simulink model "opti_debug"  (R2023a)
settings: Solver=FixedStepAuto  StartTime=0.0  StopTime=mdl.rt  RelTol=1e-3
values from neighbouring files (symbols this model uses):
  archived_Eul_XYZ = rst_Eul_XYZ.signals.values    [s4_run.m]    (also in step4_run_v1.m)
  archived_p_raw = rst_p_raw.signals.values    [s4_run.m]    (also in step4_run_v1.m)
  ctr = make_ext_tor_observer(rsim, mdl, ctr)    [s1_setup.m]    (also in setup_controller_with_functions.m = make_controller(); step1_setup.m; step1_setup_v1.m)
  ctr2 = ctr    [s1_setup.m]    (also in step1_setup.m; step1_setup_v1.m)
  lut = gen_lut    [s1_setup.m]    (also in thrust2voltage_lut_20230809.mat = ; thrust2voltage_lut_20230829.mat = )
  mdl = make_model(mdl,rsim)    [s1_setup.m]    (also in setup_controller_with_functions.m = make_model(flight_time); step1_setup.m; step1_setup_v1.m = make_model(flight_time,rsim))
  rbt = make_robot    [s1_setup.m]    (also in setup_controller_with_functions.m = make_robot(); step1_setup.m; step1_setup_v1.m)
  rbt2 = rbt    [s1_setup.m]    (also in step1_setup.m; step1_setup_v1.m)
  rsim = make_robot_simulation()    [setup_controller_with_functions.m]    (also in step1_setup_v1.m = make_simulation(rbt,mdl,rsim))
  sen = make_sensor(mdl,rsim)    [s1_setup.m]
  som = make_somersault(mdl, rsim)    [s1_setup.m]    (also in step1_setup.m)
  Time = logsout.LiveStreamSignals.getElement('voltage').Values.Time    [old_step3_run_controller_v3.m]    (also in post_identify_actuation_response.m = yout(:,1); post_thrust_torque_coefficients.m = yout(:,1))
  traj = make_trajectory(ctr, mdl, rsim)    [s1_setup.m]    (also in step1_setup.m)
undefined symbols (not defined in the file or in its folder): DiscIntNeverNeededParam, Discrete, Standard_Devices, UDP_Protocol
libraries: simulink x27, dspfdesign x12, robotcorelib x7, sldrtlib x7, slrealtimeloglib x1, shared6dof x1, dspsrcs4 x1, uavutilslib x1, ctrlSharedLib x1, dspmathops x1
(part 1 of 4)
settings Model: SimulationMode=external  ExtModeTrigDuration=5000000  Creator=SMRL  LastModifiedBy=SMRL
settings OptimizationCC: DefaultParameterBehavior=Inlined  SimCompilerOptimization=on  AccelVerboseBuild=on
settings HardwareCC: ProdBitPerLong=64  ProdHWDeviceType=Intel->x86-64 (Linux 64)
settings ModelReferenceCC: EnableParallelModelReferenceBuilds=on
settings SFSimCC: SimHardwareAcceleration=native
settings RTWCC: Description=Simulink Desktop Real-Time  SystemTargetFile=sldrt.tlc  TemplateMakefile=sldrt.tmf  RTWCompilerOptimization=on
settings CodeAppCC: MaxIdLength=95
settings SimulinkDesktopRealTimeCC: TargetLibSuffix=_sldrt.a  TargetPreCompLibLocation=C:\Program Files\MATLAB\R2023a\toolbox\sldrt\lib\win64

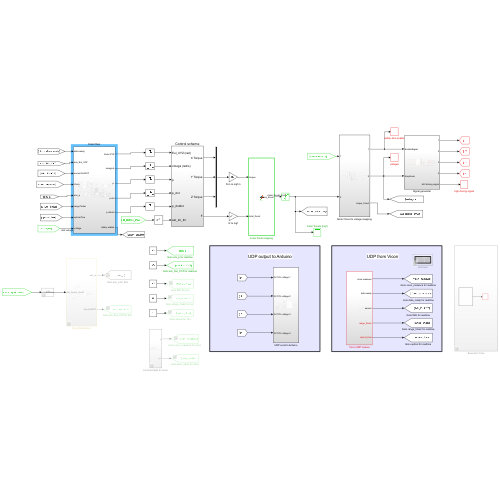
[thumbnail: Simulink's stored preview of the top-level diagram]
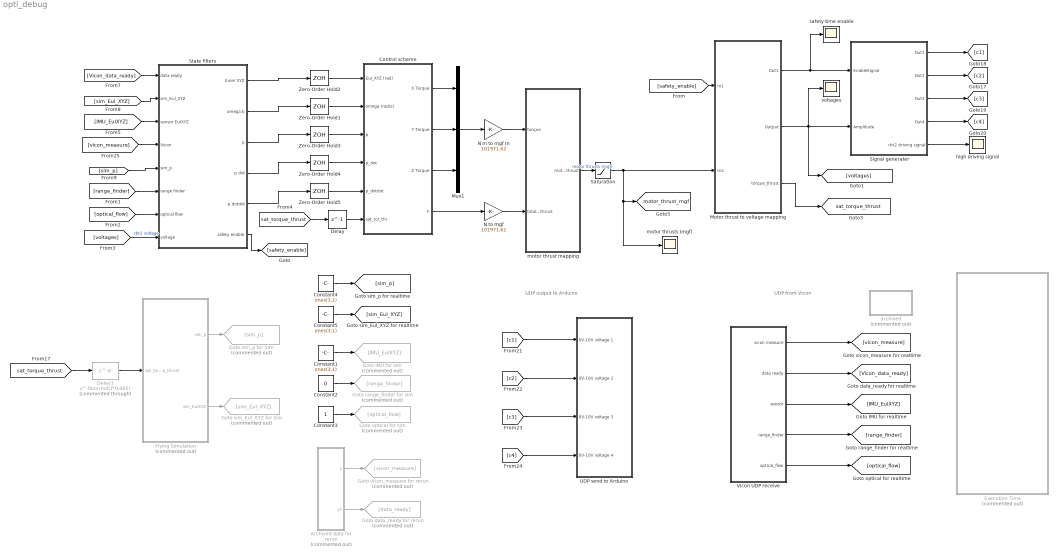
== system opti_debug ==
  note: UDP output to Arduino
  note: UDP from Vicon
  Archived data for rerun : Subsystem  Commented=on
  Constant1 : Constant  Value=ones(3,1)  SampleTime=1/400
  Constant2 : Constant  Value=0  SampleTime=1/400
  Constant3 : Constant  SampleTime=1/400
  Constant4 : Constant  Value=ones(3,1)
  Constant5 : Constant  Value=ones(3,1)
  Control scheme : Subsystem
  Delay : Delay  DelayLength=1  InitialCondition=zeros(4,1)
  Delay1 : Delay  Commented=through  DelayLength=floor(mdl.f*0.005)  InitialCondition=zeros(4,floor(mdl.f*0.005))  SampleTime=mdl.T
  Execution Time : Subsystem  Commented=on
  Flying Simulation : Subsystem  Commented=on
  Goto IMU for sim : Goto  Commented=on  GotoTag=IMU_EulXYZ
  Goto data_ready for rerun : Goto  Commented=on  GotoTag=data_ready
  Goto optical for sim : Goto  Commented=on  GotoTag=optical_flow
  Goto range_finder for sim : Goto  Commented=on  GotoTag=range_finder
  Goto sim_Eul_XYZ for Sim : Goto  Commented=on  GotoTag=sim_Eul_XYZ
  Goto sim_p for Sim : Goto  Commented=on  GotoTag=sim_p
  Goto vicon_measure for rerun : Goto  Commented=on  GotoTag=vicon_measure
  Motor thrust to voltage mapping : Subsystem
  Mux1 : Mux  Inputs=3
  N m to mgf m : Gain  Gain=101971.62
  N to mgf : Gain  Gain=101971.62
  Saturation : Saturate  UpperLimit=1000  LowerLimit=0
  Signal generater : Subsystem
  State filters : Subsystem
  UDP send to Arduino : Subsystem
  Vicon UDP receive : Subsystem
  Zero-Order Hold{1..5} (5 alike) : ZeroOrderHold  SampleTime=mdl.T
  archived : Subsystem  Commented=on
  high driving signal : Scope
  motor thrust mapping : MATLAB Function  TreatAsAtomicUnit=on  SystemSampleTime=mdl.T
  motor thrusts (mgf) : Scope
  safety-time enable : Scope
  voltages : Scope
  tag scope: motor_thrust_mgf=global, sat_torque_thrust=global
  wires:
  motor thrust mapping/1(motors_thrust) -> Saturation/1  "motor thrusts (mgf)"
  Vicon UDP receive/1(vicon measure) -> [vicon_measure]
  Vicon UDP receive/2(data ready) -> [Vicon_data_ready]
  [c1] -> UDP send to Arduino/1(0V-10V voltage 1)
  [c3] -> UDP send to Arduino/3(0V-10V voltage 3)
  [c4] -> UDP send to Arduino/4(0V-10V voltage 4)
  State filters/6(safety enable) -> [safety_enable]
  Control scheme/1(X Torque) -> Mux1/1
  Control scheme/2(Y Torque) -> Mux1/2
  Control scheme/3(Z Torque) -> Mux1/3
  [sat_torque_thrust] -> Delay1/1
  Flying Simulation/2(sim_EulXYZ) -> Goto sim_Eul_XYZ for Sim/1
  Flying Simulation/1(sim_p) -> Goto sim_p for Sim/1
  State filters/1(Euler XYZ) -> Zero-Order Hold2/1
  State filters/2(omega b) -> Zero-Order Hold1/1
  State filters/3("p ") -> Zero-Order Hold3/1
  State filters/4(p dot) -> Zero-Order Hold4/1
  Zero-Order Hold2/1 -> Control scheme/1(Eul_XYZ (rad))
  Zero-Order Hold1/1 -> Control scheme/2(omega (rad/s))
  Zero-Order Hold3/1 -> Control scheme/3(p)
  Zero-Order Hold4/1 -> Control scheme/4(p_dot)
  Zero-Order Hold5/1 -> Control scheme/5(p_dotdot)
  State filters/5(p dotdot) -> Zero-Order Hold5/1
  N m to mgf m/1 -> motor thrust mapping/1(torque)
  N to mgf/1 -> motor thrust mapping/2(total_thrust)
  Constant4/1 -> [sim_p]
  Constant5/1 -> [sim_Eul_XYZ]
  Archived data for rerun/1(y) -> Goto vicon_measure for rerun/1
  Archived data for rerun/2(y1) -> Goto data_ready for rerun/1
  Control scheme/4(" F") -> N to mgf/1
  Mux1/1 -> N m to mgf m/1
  [sat_torque_thrust] -> Delay/1
  Delay/1 -> Control scheme/6(sat_tor_thr)
  Delay1/1 -> Flying Simulation/1(sat_torque_thrust)
  Signal generater/1(Out1) -> [c1]
  Signal generater/2(Out2) -> [c2]
  Signal generater/3(Out3) -> [c3]
  Signal generater/4(Out4) -> [c4]
  Signal generater/5(rbt2 driving signal) -> high driving signal/1
  Motor thrust to voltage mapping/1(Out1) -> Signal generater/1(EnableSignal), safety-time enable/1
  [safety_enable] -> Motor thrust to voltage mapping/1(In1)
  Motor thrust to voltage mapping/2(Output) -> voltages/1, [voltages], Signal generater/2(Amplitude)
  Motor thrust to voltage mapping/3(torque_thrust) -> [sat_torque_thrust]
  Vicon UDP receive/3(sensor) -> [IMU_EulXYZ]
  [c2] -> UDP send to Arduino/2(0V-10V voltage 2)
  Vicon UDP receive/4(range_finder) -> [range_finder]
  [voltages] -> State filters/8(voltage)  "rbt2 voltage"
  [Vicon_data_ready] -> State filters/1(data ready)
  [sim_Eul_XYZ] -> State filters/2(sim_Eul_XYZ)
  [IMU_EulXYZ] -> State filters/3(sensor EulXYZ)
  [vicon_measure] -> State filters/4(Vicon)
  [sim_p] -> State filters/5(sim_p)
  [range_finder] -> State filters/6(range finder)
  Vicon UDP receive/5(optical_flow) -> [optical_flow]
  [optical_flow] -> State filters/7(optical flow)
  Constant2/1 -> Goto range_finder for sim/1
  Constant1/1 -> Goto IMU for sim/1
  Constant3/1 -> Goto optical for sim/1
  Saturation/1 -> Motor thrust to voltage mapping/2(In2), motor thrusts (mgf)/1, [motor_thrust_mgf]

== system opti_debug/Archived data for rerun ==
  MATLAB Function1 : MATLAB Function  TreatAsAtomicUnit=on
  MATLAB Function2 : MATLAB Function  TreatAsAtomicUnit=on
  Scope1 : Scope
  Scope2 : Scope
  Scope3 : Scope
  time1 : Subsystem
  y : Outport
  y1 : Outport  Port=2
  wires:
  MATLAB Function2/1(y) -> y/1, Scope1/1
  time1/1(index) -> Scope2/1, MATLAB Function2/1(t), MATLAB Function1/1(t)
  MATLAB Function1/1(y) -> y1/1, Scope3/1

== system opti_debug/Control scheme ==
  Eul_XYZ (rad) : Inport
  omega (rad/s) : Inport  Port=2
  p : Inport  Port=3
  p_dot : Inport  Port=4
  p_dotdot : Inport  Port=5
  sat_tor_thr : Inport  Port=6
  Coordinate Transformation Conversion : robotcorelib/Coordinate Transformation Conversion  InputRepresentation=Euler Angles  InputEulerSequence=XYZ  ShowTrVecInputPort=on  OutputRepresentation=Rotation Matrix  OutputEulerSequence=ZYX  ShowTrVecOutputPort=on  SimulateUsing=Interpreted execution
  Delay : Delay  DelayLength=1  InitialCondition=1
  Delay1 : Delay  DelayLength=1  InitialCondition=zeros(3,1)
  Subsystem : Subsystem
  adaptive setpoint rd : MATLAB Function  TreatAsAtomicUnit=on  SystemSampleTime=mdl.T
  all states : Scope  NumInputPorts=4
  attitude and thrust controller : Subsystem
  observer : Subsystem  Commented=on
  p vs p_des : Scope  NumInputPorts=2
  saturation : MATLAB Function  TreatAsAtomicUnit=on
  time : Subsystem
  unsat thrust : Scope
  unsat torque : Scope  NumInputPorts=3
  X Torque : Outport
  Y Torque : Outport  Port=2
  Z Torque : Outport  Port=3
  " F" : Outport  Port=4
  wires:
  Eul_XYZ (rad)/1 -> Coordinate Transformation Conversion/1
  omega (rad/s)/1 -> all states/4, attitude and thrust controller/5(Omega)
  saturation/1(X_roll) -> X Torque/1
  saturation/2(Y_pitch) -> Y Torque/1
  saturation/3(Z_yaw) -> Z Torque/1
  saturation/4(Force) -> " F"/1
  attitude and thrust controller/4(F) -> saturation/4(F), unsat thrust/1
  adaptive setpoint rd/1(rd) -> p vs p_des/2, attitude and thrust controller/6(rd)  "rd"
  adaptive setpoint rd/3(rd_dd) -> attitude and thrust controller/8(rd_dd)
  adaptive setpoint rd/4(rd_ddd) -> attitude and thrust controller/9(rd_ddd)
  adaptive setpoint rd/5(rd_dddd) -> attitude and thrust controller/10(rd_dddd)
  time/1(real times) -> adaptive setpoint rd/2(time)
  attitude and thrust controller/3(torque_z) -> saturation/3(z_yaw), unsat torque/3
  attitude and thrust controller/2(torque_y) -> saturation/2(y_pitch), unsat torque/2
  attitude and thrust controller/1(torque_x) -> unsat torque/1, saturation/1(x_roll)
  adaptive setpoint rd/7(id_out) -> Delay/1
  Delay/1 -> adaptive setpoint rd/4(id_in)
  Coordinate Transformation Conversion/1 -> all states/3, attitude and thrust controller/4(R)  "rotm"
  p_dot/1 -> all states/2, attitude and thrust controller/2(r_dot)
  p_dotdot/1 -> attitude and thrust controller/3(r_dotdot)
  p/1 -> adaptive setpoint rd/1(r), p vs p_des/1, attitude and thrust controller/1(r), all states/1
  adaptive setpoint rd/6(init_r_out) -> Delay1/1
  Delay1/1 -> adaptive setpoint rd/3(init_r_in)
  sat_tor_thr/1 -> attitude and thrust controller/11(sat_tor_thr)
  adaptive setpoint rd/2(rd_d) -> Subsystem/1(In1)
  Subsystem/1(Out1) -> attitude and thrust controller/7(rd_d)

== system opti_debug/Execution Time ==
  Execution Time : sldrtlib/Target Profiling/Execution Time  ShowTaskTimes=off
  high execution time : Scope
  wires:
  Execution Time/1 -> high execution time/1

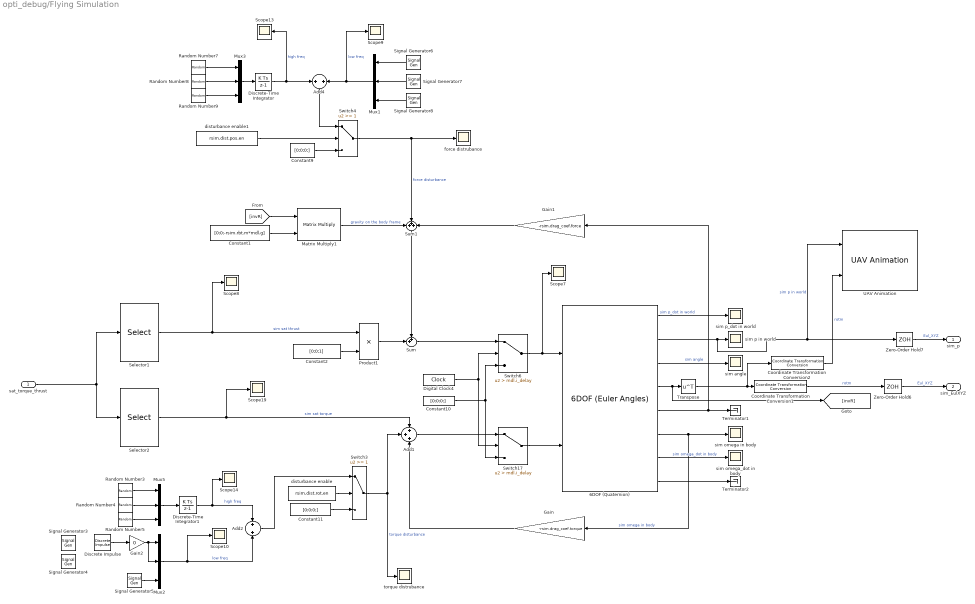
== system opti_debug/Flying Simulation ==
  sat_torque_thrust : Inport
  6DOF (Quaternion) : shared6dof/6DOF (Euler Angles)  units=Metric (MKS)  mtype=Fixed  rep=Quaternion  xme_0=rsim.p0  Vm_0=rsim.v0_b  eul_0=[rsim.Eul_XYZ.x rsim.Eul_XYZ.y rsim.Eul_XYZ.z]  pm_0=rsim.w0  mass_0=rsim.rbt.m  mass_e=0.5  mass_f=2.0  inertia=diag([rsim.rbt.ixx, rsim.rbt.iyy, rsim.rbt.izz])  inertia_e=eye(3)  inertia_f=2*eye(3)  k_quat=1.0  vre_flag=on  abi_flag=off  aMode=0  xme_statename=''  Vm_statename=''  eul_statename=''  quat_statename=''  pm_statename=''  mass_statename=''
      settings: LibrarySourceBlock=aerolib6dof2/6DOF (Quaternion)
  Add1 : Sum  Inputs=+++
  Add2 : Sum
  Add4 : Sum
  Constant1 : Constant  Value=[0;0;-rsim.rbt.m*mdl.g]
  Constant10 : Constant  Value=[0;0;0;]
  Constant11 : Constant  Value=[0;0;0;]
  Constant2 : Constant  Value=[0;0;1]
  Constant9 : Constant  Value=[0;0;0;]
  Coordinate Transformation Conversion1 : robotcorelib/Coordinate Transformation Conversion  InputRepresentation=Rotation Matrix  InputEulerSequence=XYZ  ShowTrVecInputPort=on  OutputRepresentation=Euler Angles  OutputEulerSequence=XYZ  ShowTrVecOutputPort=on  SimulateUsing=Interpreted execution
  Coordinate Transformation Conversion2 : robotcorelib/Coordinate Transformation Conversion  InputRepresentation=Rotation Matrix  InputEulerSequence=XYZ  ShowTrVecInputPort=on  OutputRepresentation=Quaternion  OutputEulerSequence=XYZ  ShowTrVecOutputPort=on  SimulateUsing=Interpreted execution
  Digital Clock4 : DigitalClock  SampleTime=1/2000
  Discrete Impulse : dspsrcs4/Discrete  Impulse  Delay=mdl.f*3.1  SampleTime=mdl.T  FrameSample=1  OutputFrames=off  dataType=double  isSigned=on  wordLen=16  udDataType=sfix(16)  fracBitsMode=Best precision  numFracBits=15  OutDataTypeStr=double  LastOutDataTypeStr=double
  Discrete-Time Integrator : DiscreteIntegrator  InitialCondition=[rsim.dist.x.mean; rsim.dist.y.mean; rsim.dist.z.mean]  SampleTime=mdl.T  ICPrevOutput=DiscIntNeverNeededParam  ICPrevScaledInput=DiscIntNeverNeededParam
  Discrete-Time Integrator1 : DiscreteIntegrator  InitialCondition=[rsim.dist.wx.mean; rsim.dist.wy.mean; rsim.dist.wz.mean]  SampleTime=mdl.T  ICPrevOutput=DiscIntNeverNeededParam  ICPrevScaledInput=DiscIntNeverNeededParam
  Gain : Gain  Gain=-rsim.drag_coef.torque
  Gain1 : Gain  Gain=-rsim.drag_coef.force
  Gain2 : Gain  Gain=0
  Matrix Multiply1 : Product  Multiplication=Matrix(*)
  Mux{1..3,5} (4 alike) : Mux  Inputs=3
  Product1 : Product
  Random Number3 : RandomNumber  Variance=rsim.dist.wx.var  Seed=rsim.dist.wx.seed  SampleTime=1/2000
  Random Number4 : RandomNumber  Variance=rsim.dist.wy.var  Seed=rsim.dist.wy.seed  SampleTime=1/2000
  Random Number5 : RandomNumber  Variance=rsim.dist.wz.var  Seed=rsim.dist.wz.seed  SampleTime=1/2000
  Random Number7 : RandomNumber  Variance=rsim.dist.x.var  Seed=rsim.dist.x.seed  SampleTime=mdl.T
  Random Number8 : RandomNumber  Variance=rsim.dist.y.var  Seed=rsim.dist.y.seed  SampleTime=mdl.T
  Random Number9 : RandomNumber  Variance=rsim.dist.z.var  Seed=rsim.dist.z.seed  SampleTime=mdl.T
  Scope{7..10,13..14,19} (7 alike) : Scope
  Selector1 : Selector  InputPortWidth=4  IndexOptions=Index vector (dialog)  Indices=[4]  OutputSizes=1
  Selector2 : Selector  InputPortWidth=4  IndexOptions=Index vector (dialog)  Indices=[1:3]  OutputSizes=1
  Signal Generator3 : SignalGenerator  WaveForm=square  Amplitude=2e-5  Frequency=0.1618
  Signal Generator4 : SignalGenerator  WaveForm=square  Amplitude=0e-5  Frequency=0.162
  Signal Generator5 : SignalGenerator  Amplitude=-30e-8  Frequency=0.4
  Signal Generator6 : SignalGenerator  WaveForm=square  Amplitude=0  Frequency=0.1
  Signal Generator7 : SignalGenerator  WaveForm=square  Amplitude=0  Frequency=0.5
  Signal Generator8 : SignalGenerator  WaveForm=square  Amplitude=0  Frequency=0.5
  Sum : Sum  Inputs=++|
  Sum1 : Sum  Inputs=+++
  Switch17 : Switch  Criteria=u2 > Threshold  Threshold=mdl.i_delay  SaturateOnIntegerOverflow=off  InputSameDT=off
  Switch3 : Switch  Threshold=1  SaturateOnIntegerOverflow=off  InputSameDT=off
  Switch4 : Switch  Threshold=1  SaturateOnIntegerOverflow=off  InputSameDT=off
  Switch6 : Switch  Criteria=u2 > Threshold  Threshold=mdl.i_delay  SaturateOnIntegerOverflow=off  InputSameDT=off
  Terminator1 : Terminator
  Terminator2 : Terminator
  Transpose : Math  Operator=transpose  SignedPower=on
  UAV Animation : uavutilslib/UAV Animation  UAVType=Multirotor  UAVSize=0.1  InertialZDirection=Up  SampleTime=1/100
  Zero-Order Hold6 : ZeroOrderHold  SampleTime=1/400
  Zero-Order Hold7 : ZeroOrderHold  SampleTime=1/400
  disturbance enable : Constant  Value=rsim.dist.rot.en
  disturbance enable1 : Constant  Value=rsim.dist.pos.en
  force distrubance : Scope
  sim angle : Scope
  sim omega in body : Scope
  sim omega_dot in body : Scope
  sim p in world : Scope
  sim p_dot in world : Scope
  torque distrubance : Scope
  sim_p : Outport
  sim_EulXYZ : Outport  Port=2
  wires:
  Random Number5/1 -> Mux5/3
  disturbance enable/1 -> Switch3/2
  Mux5/1 -> Discrete-Time Integrator1/1
  Digital Clock4/1 -> Switch6/2, Switch17/2
  Constant11/1 -> Switch3/3
  Constant2/1 -> Product1/2
  Constant1/1 -> Matrix Multiply1/2
  Random Number3/1 -> Mux5/1
  Matrix Multiply1/1 -> Sum1/1  "gravity on the body frame"
  disturbance enable1/1 -> Switch4/2
  Random Number4/1 -> Mux5/2
  Switch3/1 -> Add1/2, torque distrubance/1  "torque disturbance"
  Constant9/1 -> Switch4/3
  [invR] -> Matrix Multiply1/1
  Constant10/1 -> Switch6/3, Switch17/3
  Sum1/1 -> Sum/1
  Sum/1 -> Switch6/1
  Switch4/1 -> Sum1/2, force distrubance/1  "force disturbance"
  Product1/1 -> Sum/2
  Add1/1 -> Switch17/1
  Switch6/1 -> Scope7/1, 6DOF (Quaternion)/1
  Switch17/1 -> 6DOF (Quaternion)/2
  6DOF (Quaternion)/1 -> sim p_dot in world/1  "sim p_dot in world"
  6DOF (Quaternion)/2 -> UAV Animation/1, Zero-Order Hold7/1, sim p in world/1  "sim p in world"
  6DOF (Quaternion)/3 -> sim angle/1  "sim angle"
  6DOF (Quaternion)/4 -> [invR], Transpose/1
  6DOF (Quaternion)/5 -> Gain1/1, Terminator1/1
  6DOF (Quaternion)/6 -> Gain/1, sim omega in body/1  "sim omega in body"
  6DOF (Quaternion)/7 -> sim omega_dot in body/1  "sim omega_dot in body"
  6DOF (Quaternion)/8 -> Terminator2/1
  Transpose/1 -> Coordinate Transformation Conversion2/1, Coordinate Transformation Conversion1/1
  Zero-Order Hold6/1 -> sim_EulXYZ/1  "Eul_XYZ"
  Coordinate Transformation Conversion1/1 -> Zero-Order Hold6/1  "rotm"
  Zero-Order Hold7/1 -> sim_p/1  "Eul_XYZ"
  Mux2/1 -> Scope10/1, Add2/2  "low freq"
  Signal Generator5/1 -> Mux2/3
  sat_torque_thrust/1 -> Selector1/1, Selector2/1
  Selector1/1 -> Scope8/1, Product1/1  "sim sat thrust"
  Selector2/1 -> Scope19/1, Add1/1  "sim sat torque"
  Random Number7/1 -> Mux3/1
  Mux3/1 -> Discrete-Time Integrator/1
  Random Number8/1 -> Mux3/2
  Random Number9/1 -> Mux3/3
  Discrete-Time Integrator/1 -> Add4/1, Scope13/1  "high freq"
  Mux1/1 -> Scope9/1, Add4/2  "low freq"
  Signal Generator8/1 -> Mux1/3
  Signal Generator7/1 -> Mux1/2
  Signal Generator6/1 -> Mux1/1
  Add4/1 -> Switch4/1
  Discrete-Time Integrator1/1 -> Add2/1, Scope14/1  "high freq"
  Add2/1 -> Switch3/1
  Coordinate Transformation Conversion2/1 -> UAV Animation/2  "rotm"
  Gain/1 -> Add1/3
  Gain1/1 -> Sum1/3
  Discrete Impulse/1 -> Gain2/1
  Gain2/1 -> Mux2/2, Mux2/1

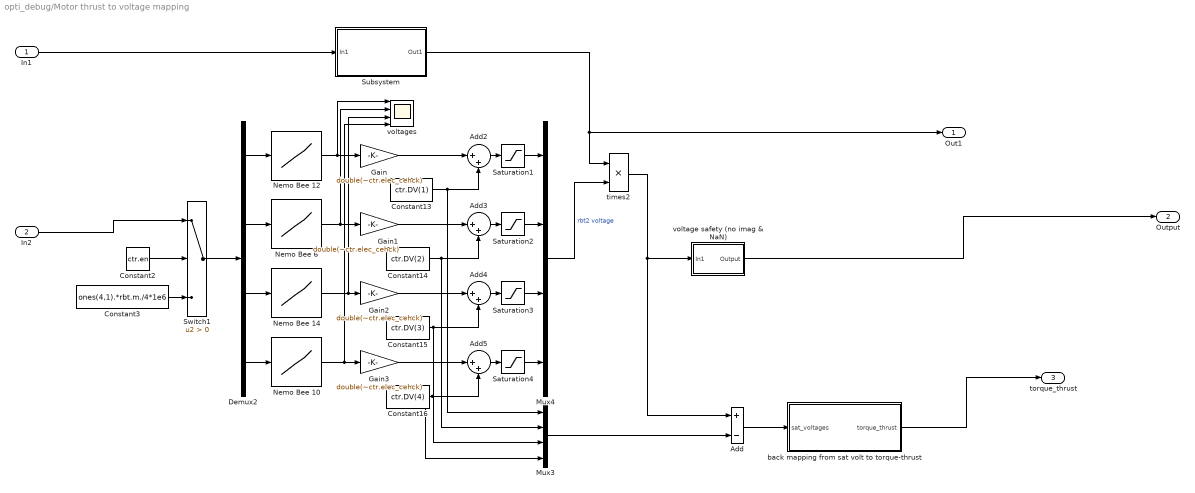
== system opti_debug/Motor thrust to voltage mapping ==
  In1 : Inport
  In2 : Inport  Port=2
  Add : Sum  Inputs=+-
  Add{2..5} (4 alike) : Sum  Inputs=|++
  Constant13 : Constant  Value=ctr.DV(1)
  Constant14 : Constant  Value=ctr.DV(2)
  Constant15 : Constant  Value=ctr.DV(3)
  Constant16 : Constant  Value=ctr.DV(4)
  Constant2 : Constant  Value=ctr.en
  Constant3 : Constant  Value=ones(4,1).*rbt.m./4*1e6
  Demux2 : Demux
  Gain{,1..3} (4 alike) : Gain  Gain=double(~ctr.elec_cehck)
  Mux3 : Mux
  Mux4 : Mux
  Nemo Bee 10 : Lookup_n-D  NumberOfTableDimensions=1  BreakpointsForDimension1=lut.T4  Table=lut.v4  InternalRulePriority=Speed  RndMeth=Simplest
  Nemo Bee 12 : Lookup_n-D  NumberOfTableDimensions=1  BreakpointsForDimension1=lut.T1  Table=lut.v1  InternalRulePriority=Speed  RndMeth=Simplest
  Nemo Bee 14 : Lookup_n-D  NumberOfTableDimensions=1  BreakpointsForDimension1=lut.T3  Table=lut.v3  InternalRulePriority=Speed  RndMeth=Simplest
  Nemo Bee 6 : Lookup_n-D  NumberOfTableDimensions=1  BreakpointsForDimension1=lut.T2  Table=lut.v2  InternalRulePriority=Speed  RndMeth=Simplest
  Saturation1 : Saturate  UpperLimit=ctr.safety.volt(1)  LowerLimit=0
  Saturation2 : Saturate  UpperLimit=ctr.safety.volt(2)  LowerLimit=0
  Saturation3 : Saturate  UpperLimit=ctr.safety.volt(3)  LowerLimit=0
  Saturation4 : Saturate  UpperLimit=ctr.safety.volt(4)  LowerLimit=0
  Subsystem : Subsystem
  Switch1 : Switch  Criteria=u2 > Threshold  SaturateOnIntegerOverflow=off  InputSameDT=off
  back mapping from sat volt to torque-thrust : Subsystem
  times2 : Product  RndMeth=Zero
  voltage safety (no imag & NaN) : Subsystem
  voltages : Scope  NumInputPorts=4
  Out1 : Outport
  Output : Outport  Port=2
  torque_thrust : Outport  Port=3
  wires:
  Add4/1 -> Saturation3/1
  Nemo Bee 6/1 -> voltages/2, Gain1/1
  Gain1/1 -> Add3/1
  Add2/1 -> Saturation1/1
  Saturation4/1 -> Mux4/4
  Demux2/1 -> Nemo Bee 12/1
  Constant3/1 -> Switch1/3
  In2/1 -> Switch1/1
  Add5/1 -> Saturation4/1
  Add/1 -> back mapping from sat volt to torque-thrust/1(sat_voltages)
  Gain/1 -> Add2/1
  Constant2/1 -> Switch1/2
  Nemo Bee 12/1 -> voltages/1, Gain/1
  Mux3/1 -> Add/2
  Constant13/1 -> Mux3/1, Add2/2
  Saturation2/1 -> Mux4/2
  Nemo Bee 10/1 -> voltages/4, Gain3/1
  back mapping from sat volt to torque-thrust/1(torque_thrust) -> torque_thrust/1
  Demux2/2 -> Nemo Bee 6/1
  Constant14/1 -> Mux3/2, Add3/2
  Mux4/1 -> times2/2  "rbt2 voltage"
  Demux2/4 -> Nemo Bee 10/1
  Add3/1 -> Saturation2/1
  times2/1 -> Add/1, voltage safety (no imag & NaN)/1(In1)
  In1/1 -> Subsystem/1(In1)
  Switch1/1 -> Demux2/1
  Constant16/1 -> Mux3/4, Add5/2
  Demux2/3 -> Nemo Bee 14/1
  Nemo Bee 14/1 -> voltages/3, Gain2/1
  Subsystem/1(Out1) -> Out1/1, times2/1
  Gain3/1 -> Add5/1
  Gain2/1 -> Add4/1
  Constant15/1 -> Mux3/3, Add4/2
  Saturation3/1 -> Mux4/3
  Saturation1/1 -> Mux4/1
  voltage safety (no imag & NaN)/1(Output) -> Output/1

== system opti_debug/Signal generater ==
  EnableSignal : Inport
  Amplitude : Inport  Port=2
  Demux4 : Demux
  Flapping Freq (Hz) : Constant  Value=ctr.freq_vec  VectorParams1D=off  SampleTime=mdl.T_high
  Mux7 : Mux
  c1 (JP1) : Gain  Gain=0.9739
  c2 (B1) : Gain  Gain=0.9947
  c3 (W1)1 : Gain  Gain=0.9769
  c4 (JP2) : Gain  Gain=0.9910
  safety voltage : Constant  Value=ctr.safety.volt  SampleTime=mdl.T_high
  signal generator1 : Subsystem  SystemSampleTime=mdl.T_high
  signal safety (no imag & NaN) : Subsystem
  Out1 : Outport
  Out2 : Outport  Port=2
  Out3 : Outport  Port=3
  Out4 : Outport  Port=4
  rbt2 driving signal : Outport  Port=5
  wires:
  Mux7/1 -> rbt2 driving signal/1, signal safety (no imag & NaN)/1(In1)  "rbt2 driving signal"
  signal generator1/1(D2A DriveSignal 1) -> Mux7/1
  safety voltage/1 -> signal generator1/2(safety voltage)
  signal safety (no imag & NaN)/1(Output) -> Demux4/1
  Demux4/3 -> c3 (W1)1/1
  Demux4/1 -> c1 (JP1)/1
  Demux4/2 -> c2 (B1)/1
  signal generator1/2(D2A DriveSignal 2) -> Mux7/2
  Demux4/4 -> c4 (JP2)/1
  Flapping Freq (Hz)/1 -> signal generator1/3(frequency_vec (hz))
  signal generator1/3(D2A DriveSignal 3) -> Mux7/3
  signal generator1/4(D2A DriveSignal 4) -> Mux7/4
  EnableSignal/1 -> signal generator1/1(EnableSignal)
  c4 (JP2)/1 -> Out4/1
  c1 (JP1)/1 -> Out1/1
  c2 (B1)/1 -> Out2/1
  c3 (W1)1/1 -> Out3/1
  Amplitude/1 -> signal generator1/4(Amplitude)

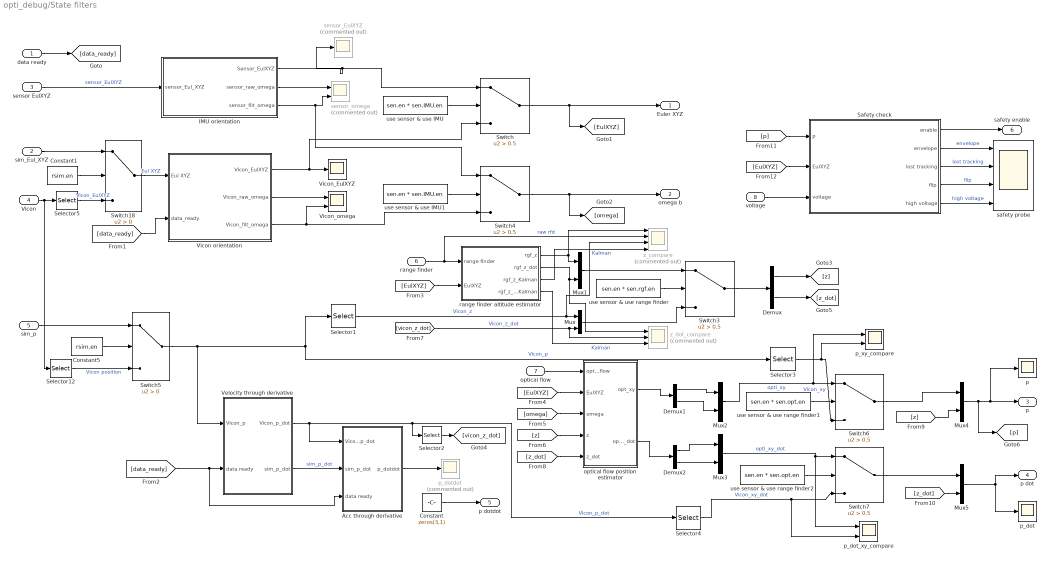
== system opti_debug/State filters ==
  data ready : Inport
  sim_Eul_XYZ : Inport  Port=2
  sensor EulXYZ : Inport  Port=3
  Vicon : Inport  Port=4
  sim_p : Inport  Port=5
  range finder : Inport  Port=6
  optical flow : Inport  Port=7
  voltage : Inport  Port=8
  Acc through derivative : Subsystem
  Constant : Constant  Value=zeros(3,1)
  Constant1 : Constant  Value=rsim.en
  Constant5 : Constant  Value=rsim.en
  Demux : Demux  Outputs=2
  Demux1 : Demux  Outputs=2
  Demux2 : Demux  Outputs=2
  IMU orientation : Subsystem
  Mux{,1..5} (6 alike) : Mux  Inputs=2
  Safety check : Subsystem  SystemSampleTime=mdl.T
  Selector1 : Selector  InputPortWidth=3  IndexOptions=Index vector (dialog)  Indices=[3]  OutputSizes=1
  Selector12 : Selector  InputPortWidth=6  IndexOptions=Index vector (dialog)  Indices=[1:3]  OutputSizes=1
  Selector2 : Selector  InputPortWidth=3  IndexOptions=Index vector (dialog)  Indices=[3]  OutputSizes=1
  Selector3 : Selector  InputPortWidth=3  IndexOptions=Index vector (dialog)  Indices=[1 2]  OutputSizes=1
  Selector4 : Selector  InputPortWidth=3  IndexOptions=Index vector (dialog)  Indices=[1 2]  OutputSizes=1
  Selector5 : Selector  InputPortWidth=6  IndexOptions=Index vector (dialog)  Indices=[4:6]  OutputSizes=1
  Switch{,3..4,6..7} (5 alike) : Switch  Criteria=u2 > Threshold  Threshold=0.5  SaturateOnIntegerOverflow=off  InputSameDT=off
  Switch18 : Switch  Criteria=u2 > Threshold  SaturateOnIntegerOverflow=off  InputSameDT=off
  Switch5 : Switch  Criteria=u2 > Threshold  SaturateOnIntegerOverflow=off  InputSameDT=off
  Velocity through derivative : Subsystem
  Vicon orientation : Subsystem
  Vicon_EulXYZ : Scope
  Vicon_omega : Scope  NumInputPorts=2
  optical flow position estimator : Subsystem
  p : Scope
  p_dot : Scope
  p_dot_xy_compare : Scope  NumInputPorts=2
  p_dotdot : Scope  Commented=on
  p_xy_compare : Scope  NumInputPorts=2
  range finder altitude estimator : Subsystem
  safety probe : Scope  NumInputPorts=4
  sensor_EulXYZ : Scope  Commented=on
  sensor_omega : Scope  Commented=on  NumInputPorts=2
  use sensor & use IMU : Constant  Value=sen.en * sen.IMU.en
  use sensor & use IMU1 : Constant  Value=sen.en * sen.IMU.en
  use sensor & use range finder : Constant  Value=sen.en * sen.rgf.en
  use sensor & use range finder1 : Constant  Value=sen.en * sen.opt.en
  use sensor & use range finder2 : Constant  Value=sen.en * sen.opt.en
  z_compare : Scope  Commented=on  NumInputPorts=4
  z_dot_compare : Scope  Commented=on  NumInputPorts=3
  Euler XYZ : Outport
  omega b : Outport  Port=2
  "p " : Outport  Port=3
  p dot : Outport  Port=4
  p dotdot : Outport  Port=5
  safety enable : Outport  Port=6
  wires:
  Switch5/1 -> Velocity through derivative/1(Vicon_p), Selector1/1, Selector3/1  "Vicon_p"
  Constant1/1 -> Switch18/2
  Vicon/1 -> Selector12/1, Selector5/1
  data ready/1 -> [data_ready]
  sim_p/1 -> Switch5/1
  sim_Eul_XYZ/1 -> Switch18/1
  Safety check/1(enable) -> safety enable/1
  Safety check/2(envelope) -> safety probe/1  "envelope"
  Safety check/3(lost tracking) -> safety probe/2  "lost tracking"
  Safety check/4(flip) -> safety probe/3  "flip"
  Safety check/5(high voltage) -> safety probe/4  "high voltage"
  voltage/1 -> Safety check/3(voltage)
  use sensor & use IMU/1 -> Switch/2
  Switch/1 -> [EulXYZ], Euler XYZ/1
  Switch4/1 -> omega b/1, [omega]
  use sensor & use IMU1/1 -> Switch4/2
  Constant5/1 -> Switch5/2
  range finder/1 -> range finder altitude estimator/1(range finder), z_compare/2  "raw rfd"
  optical flow/1 -> optical flow position estimator/1(optical flow)
  optical flow position estimator/1(opt_xy) -> Demux1/1
  [EulXYZ] -> range finder altitude estimator/2(EulXYZ)
  use sensor & use range finder/1 -> Switch3/2
  [EulXYZ] -> optical flow position estimator/2(EulXYZ)
  [omega] -> optical flow position estimator/3(omega)
  optical flow position estimator/2(opt_xy_dot) -> Demux2/1
  Selector2/1 -> [vicon_z_dot]
  [vicon_z_dot] -> z_dot_compare/2, Mux/2  "Vicon_z_dot"
  Selector1/1 -> z_compare/3, Mux/1  "Vicon_z"
  Mux/1 -> Switch3/3
  range finder altitude estimator/1(rgf_z) -> z_compare/1, Mux1/1
  range finder altitude estimator/2(rgf_z_dot) -> z_dot_compare/1, Mux1/2
  Mux1/1 -> Switch3/1
  Switch3/1 -> Demux/1
  Demux/1 -> [z]
  Demux/2 -> [z_dot]
  [z] -> optical flow position estimator/4(z)
  Demux1/1 -> Mux2/1
  Demux1/2 -> Mux2/2
  Demux2/2 -> Mux3/2
  Demux2/1 -> Mux3/1
  use sensor & use range finder1/1 -> Switch6/2
  Mux2/1 -> p_xy_compare/1, Switch6/1  "opti_xy"
  use sensor & use range finder2/1 -> Switch7/2
  Mux3/1 -> p_dot_xy_compare/1, Switch7/1  "opti_xy_dot"
  Mux5/1 -> p dot/1, p_dot/1
  [p] -> Safety check/1(p)
  [EulXYZ] -> Safety check/2(EulXYZ)
  IMU orientation/1(Sensor_EulXYZ) -> Switch/1, sensor_EulXYZ/1
  IMU orientation/3(sensor_filt_omega) -> sensor_omega/2, Switch4/1
  sensor EulXYZ/1 -> IMU orientation/1(sensor_Eul_XYZ)  "sensor_EulXYZ"
  IMU orientation/2(sensor_raw_omega) -> sensor_omega/1
  Vicon orientation/1(Vicon_EulXYZ) -> Switch/3, Vicon_EulXYZ/1
  Vicon orientation/3(Vicon_filt_omega) -> Switch4/3, Vicon_omega/2
  Switch18/1 -> Vicon orientation/1(Eul XYZ)  "Eul XYZ"
  Vicon orientation/2(Vicon_raw_omega) -> Vicon_omega/1
  Constant/1 -> p dotdot/1
  Velocity through derivative/1(Vicon_p_dot) -> Selector4/1, Selector2/1, Acc through derivative/1(Vicon_p_dot)  "Vicon_p_dot"
  [data_ready] -> Acc through derivative/3(data ready), Velocity through derivative/2(data ready)
  Velocity through derivative/2(sim_p_dot) -> Acc through derivative/2(sim_p_dot)  "sim_p_dot"
  Acc through derivative/1(p_dotdot) -> p_dotdot/1
  [data_ready] -> Vicon orientation/2(data_ready)
  Selector3/1 -> p_xy_compare/2, Switch6/3  "Vicon_xy"
  [z] -> Mux4/2
  Switch6/1 -> Mux4/1
  Mux4/1 -> [p], "p "/1, p/1
  Selector4/1 -> p_dot_xy_compare/2, Switch7/3  "Vicon_xy_dot"
  [z_dot] -> Mux5/2
  Switch7/1 -> Mux5/1
  range finder altitude estimator/3(rgf_z_Kalman) -> z_compare/4  "Kalman"
  range finder altitude estimator/4(rgf_z_dot_Kalman) -> z_dot_compare/3  "Kalman"
  Selector12/1 -> Switch5/3  "Vicon position"
  Selector5/1 -> Switch18/3  "Vicon_EulXYZ"
  [z_dot] -> optical flow position estimator/5(z_dot)

== system opti_debug/UDP send to Arduino ==
  0V-10V voltage 1 : Inport
  0V-10V voltage 2 : Inport  Port=2
  0V-10V voltage 3 : Inport  Port=3
  0V-10V voltage 4 : Inport  Port=4
  Digital Clock : DigitalClock  SampleTime=1/10000
  Packet Output : sldrtlib/Packet Output  SampleTime=1/10000  MaxMissedTicks=100  ShowMissedTicks=off  YieldWhenWaiting=off  DrvName=Standard_Devices/UDP_Protocol  DrvAddress=22099  DrvOptions=[0 25000 49 54 57 46 50 53 52 46 49 48 51 46 52 50 0 0 0 0 0 0 0 0 0 0 0 0 0 0 0 0 0 0 0 0 0 0 0 0 0 0 0 0 0 0 0 0 0 0 0 0 0 0 0 0 0 0 0 0 0 0 0 0 0 0 0 0 0 0 0 0 0 0 0 0 0 0 0 0 0 0 0 0 0 0 0 0 0 0 0 0 0 0 0 0 0 0 0 0 0 0 0 0 0 0 0 0 0 0 0 0 0 0 0 0 0 0 0 0 0 0 0 0 0 0 0 0 0 0 0 0 0 0 0 0 0 0 0 0 0 0 0 0 0 0 0 0 0 0 0 0 0 0 0 0 0 0 0 0 0 0 0 0 0 0 0 0 0 0 0 0 0 0 0 0 0 0 0 0 0 0 0 0 0 0 0 0 0 0 0 0 0 0 0 0 0 0 0 0 0 0 0 0 0 0 0 0 0 0 0 0 0 0 0 0 0 0 0 0 0 0 0 0 0 0 0 0 0 0 0 0 0 0 0 0 0 0 0 0 0 0 0 0 0 0 0 0 0 0 0 0 0 0 0 0]  PacketSize=8  DataTypes='4*uint16'  ShowReady=off  ShowError=off  PacketID=1  ByteOrder=1  InitialValue=[]  FinalValue=[]
      settings: AttributesFormatString=UDP Protocol [22099]
  Switch : Switch  Criteria=u2 > Threshold  Threshold=2  SaturateOnIntegerOverflow=off  InputSameDT=off
  UDP send to Arduino DAC : Subsystem
  constant1 : Constant  Value=0  OutDataTypeStr=boolean
  constant2 : Constant  OutDataTypeStr=boolean
  wires:
  UDP send to Arduino DAC/1(Output) -> Packet Output/1
  0V-10V voltage 2/1 -> UDP send to Arduino DAC/2(DAC2)
  0V-10V voltage 4/1 -> UDP send to Arduino DAC/4(DAC4)
  0V-10V voltage 1/1 -> UDP send to Arduino DAC/1(DAC1)
  Switch/1 -> UDP send to Arduino DAC/5(DO2)
  0V-10V voltage 3/1 -> UDP send to Arduino DAC/3(DAC3)
  constant1/1 -> Switch/1
  constant2/1 -> Switch/3
  Digital Clock/1 -> Switch/2

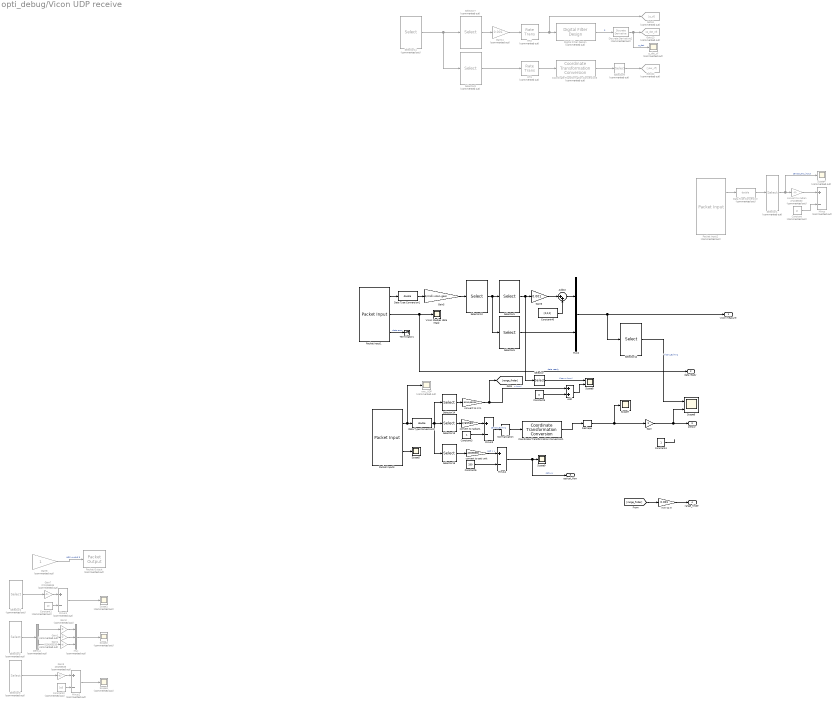
== system opti_debug/Vicon UDP receive ==
  Add : Sum
  Add10 : Sum  Inputs=|++
  Constant : Constant  Commented=on  Value=pi
  Constant1 : Constant  Commented=on  Value=10
  Constant2 : Constant  Commented=on  Value=1e3
  Constant3 : Constant
  Constant4 : Constant
  Constant40 : Constant  Value=[0,0,0]
  Constant5 : Constant  Value=0
  Constant6 : Constant  Value=200
  Coordinate Transformation Conversion1 : robotcorelib/Coordinate Transformation Conversion  InputRepresentation=Quaternion  InputEulerSequence=XYZ  ShowTrVecInputPort=on  OutputRepresentation=Euler Angles  OutputEulerSequence=XYZ  ShowTrVecOutputPort=on  SimulateUsing=Code generation
  Coordinate Transformation Conversion3 : robotcorelib/Coordinate Transformation Conversion  Commented=on  InputRepresentation=Euler Angles  InputEulerSequence=XYZ  ShowTrVecInputPort=on  OutputRepresentation=Euler Angles  OutputEulerSequence=ZYX  ShowTrVecOutputPort=on  SimulateUsing=Interpreted execution
  Data Type Conversion : DataTypeConversion  Commented=on  OutDataTypeStr=double  SaturateOnIntegerOverflow=off  RndMeth=Floor
  Data Type Conversion1 : DataTypeConversion  OutDataTypeStr=double  SaturateOnIntegerOverflow=off  RndMeth=Floor
  Data Type Conversion2 : DataTypeConversion  OutDataTypeStr=double  SaturateOnIntegerOverflow=off  RndMeth=Floor
  Demux : Demux  Commented=on  Outputs=3
  Digital Filter Design : dspfdesign/Digital Filter Design  Commented=on  mwdsp_browser_bugfix_var=off
  Discrete Derivative2 : simulink/Discrete/Discrete Derivative  Commented=on  gainval=1.0  ICPrevScaledInput=0.0  OutMin=[]  OutMax=[]  OutDataType=fixdt(1, 16)  OutScaling=2^-10  DoSatur=off
  Gain : Gain
  Gain1 : Gain  Commented=on  Gain=0
  Gain11 : Gain  Commented=on  Gain=0.001
  Gain2 : Gain  Commented=on  Gain=0
  Gain3 : Gain  Commented=on  Gain=2e3/65535
  Gain4 : Gain  Commented=on  Gain=8190/65535
  Gain5 : Gain  Gain=1/mdl.vicon.gain
  Gain6 : Gain  Gain=0.001
  Gain7 : Gain  Commented=on  Gain=2*10/65535
  Gain8 : Gain  Commented=on  OutDataTypeStr=uint16
  Goto13 : Goto  Commented=on  GotoTag=p_dot_cf
  Goto22 : Goto  Commented=on  GotoTag=yaw_cf
  Goto3 : Goto  Commented=on  GotoTag=p_cf
  Minus : Sum  Commented=on  Inputs=+-
  Minus1 : Sum  Commented=on  Inputs=+-
  Minus2 : Sum  Commented=on  Inputs=+-
  Minus3 : Sum  Inputs=+-
  Minus4 : Sum  Inputs=+-
  Mux : Mux  Commented=on  Inputs=3
  Mux2 : Mux  Inputs=2
  Normalization : dspmathops/Normalization  NormType=Squared 2-norm  Bias=1e-10  NormOver=Each column  Dimension=1  roundingMode=Floor  overflowMode=off  accumDataTypeStr=Inherit: Same as product output  accumLastDataTypeStr=Inherit: Same as product output  outputDataTypeStr=Inherit: Same as product output  outputMin=[]  outputMax=[]  outputLastDataTypeStr=Inherit: Same as product output
  Packet Input1 : sldrtlib/Packet Input  SampleTime=1/10000  MaxMissedTicks=100  ShowMissedTicks=off  YieldWhenWaiting=on  DrvName=Standard_Devices/UDP_Protocol  DrvAddress=18000  DrvOptions=[0 18885 49 54 57 46 50 53 52 46 49 54 56 46 49 52 54 0 0 0 0 0 0 0 0 0 0 0 0 0 0 0 0 0 0 0 0 0 0 0 0 0 0 0 0 0 0 0 0 0 0 0 0 0 0 0 0 0 0 0 0 0 0 0 0 0 0 0 0 0 0 0 0 0 0 0 0 0 0 0 0 0 0 0 0 0 0 0 0 0 0 0 0 0 0 0 0 0 0 0 0 0 0 0 0 0 0 0 0 0 0 0 0 0 0 0 0 0 0 0 0 0 0 0 0 0 0 0 0 0 0 0 0 0 0 0 0 0 0 0 0 0 0 0 0 0 0 0 0 0 0 0 0 0 0 0 0 0 0 0 0 0 0 0 0 0 0 0 0 0 0 0 0 0 0 0 0 0 0 0 0 0 0 0 0 0 0 0 0 0 0 0 0 0 0 0 0 0 0 0 0 0 0 0 0 0 0 0 0 0 0 0 0 0 0 0 0 0 0 0 0 0 0 0 0 0 0 0 0 0 0 0 0 0 0 0 0 0 0 0 0 0 0 0 0 0 0 0 0 0 0 0 0 0 0 0]  PacketSize=48  DataTypes='12*int32'  ShowReady=on  ShowError=on  PacketID=1  ByteOrder=2  ShowTimestamp=off
      settings: AttributesFormatString=UDP Protocol [18000]
  Packet Input2 : sldrtlib/Packet Input  Commented=on  SampleTime=1/10000  MaxMissedTicks=100  ShowMissedTicks=off  YieldWhenWaiting=on  DrvName=Standard_Devices/UDP_Protocol  DrvAddress=1500  DrvOptions=[0 16385 49 57 50 46 49 54 56 46 55 46 51 0 0 0 0 0 0 0 0 0 0 0 0 0 0 0 0 0 0 0 0 0 0 0 0 0 0 0 0 0 0 0 0 0 0 0 0 0 0 0 0 0 0 0 0 0 0 0 0 0 0 0 0 0 0 0 0 0 0 0 0 0 0 0 0 0 0 0 0 0 0 0 0 0 0 0 0 0 0 0 0 0 0 0 0 0 0 0 0 0 0 0 0 0 0 0 0 0 0 0 0 0 0 0 0 0 0 0 0 0 0 0 0 0 0 0 0 0 0 0 0 0 0 0 0 0 0 0 0 0 0 0 0 0 0 0 0 0 0 0 0 0 0 0 0 0 0 0 0 0 0 0 0 0 0 0 0 0 0 0 0 0 0 0 0 0 0 0 0 0 0 0 0 0 0 0 0 0 0 0 0 0 0 0 0 0 0 0 0 0 0 0 0 0 0 0 0 0 0 0 0 0 0 0 0 0 0 0 0 0 0 0 0 0 0 0 0 0 0 0 0 0 0 0 0 0 0 0 0 0 0 0 0 0 0 0 0 0 0 0 0 0 0 0]  PacketSize=6  DataTypes='3*uint16'  ShowReady=on  ShowError=off  PacketID=1  ByteOrder=1  ShowTimestamp=off
      settings: AttributesFormatString=UDP Protocol [1500]
  Packet Input3 : sldrtlib/Packet Input  SampleTime=1/10000  MaxMissedTicks=100  ShowMissedTicks=off  YieldWhenWaiting=on  DrvName=Standard_Devices/UDP_Protocol  DrvAddress=1500  DrvOptions=[0 16385 49 57 50 46 49 54 56 46 55 46 51 0 0 0 0 0 0 0 0 0 0 0 0 0 0 0 0 0 0 0 0 0 0 0 0 0 0 0 0 0 0 0 0 0 0 0 0 0 0 0 0 0 0 0 0 0 0 0 0 0 0 0 0 0 0 0 0 0 0 0 0 0 0 0 0 0 0 0 0 0 0 0 0 0 0 0 0 0 0 0 0 0 0 0 0 0 0 0 0 0 0 0 0 0 0 0 0 0 0 0 0 0 0 0 0 0 0 0 0 0 0 0 0 0 0 0 0 0 0 0 0 0 0 0 0 0 0 0 0 0 0 0 0 0 0 0 0 0 0 0 0 0 0 0 0 0 0 0 0 0 0 0 0 0 0 0 0 0 0 0 0 0 0 0 0 0 0 0 0 0 0 0 0 0 0 0 0 0 0 0 0 0 0 0 0 0 0 0 0 0 0 0 0 0 0 0 0 0 0 0 0 0 0 0 0 0 0 0 0 0 0 0 0 0 0 0 0 0 0 0 0 0 0 0 0 0 0 0 0 0 0 0 0 0 0 0 0 0 0 0 0 0 0 0]  PacketSize=14  DataTypes='7*uint16'  ShowReady=on  ShowError=off  PacketID=1  ByteOrder=1  ShowTimestamp=off
      settings: AttributesFormatString=UDP Protocol [1500]
  Packet Output : sldrtlib/Packet Output  Commented=on  SampleTime=1/10000  MaxMissedTicks=100  ShowMissedTicks=off  YieldWhenWaiting=off  DrvName=Standard_Devices/UDP_Protocol  DrvAddress=1997  DrvOptions=[0 16388 49 57 50 46 49 54 56 46 55 46 51 0 0 0 0 0 0 0 0 0 0 0 0 0 0 0 0 0 0 0 0 0 0 0 0 0 0 0 0 0 0 0 0 0 0 0 0 0 0 0 0 0 0 0 0 0 0 0 0 0 0 0 0 0 0 0 0 0 0 0 0 0 0 0 0 0 0 0 0 0 0 0 0 0 0 0 0 0 0 0 0 0 0 0 0 0 0 0 0 0 0 0 0 0 0 0 0 0 0 0 0 0 0 0 0 0 0 0 0 0 0 0 0 0 0 0 0 0 0 0 0 0 0 0 0 0 0 0 0 0 0 0 0 0 0 0 0 0 0 0 0 0 0 0 0 0 0 0 0 0 0 0 0 0 0 0 0 0 0 0 0 0 0 0 0 0 0 0 0 0 0 0 0 0 0 0 0 0 0 0 0 0 0 0 0 0 0 0 0 0 0 0 0 0 0 0 0 0 0 0 0 0 0 0 0 0 0 0 0 0 0 0 0 0 0 0 0 0 0 0 0 0 0 0 0 0 0 0 0 0 0 0 0 0 0 0 0 0 0 0 0 0 0 0]  PacketSize=2  DataTypes='1*uint16'  ShowReady=off  ShowError=off  PacketID=1  ByteOrder=1  InitialValue=1  FinalValue=1
      settings: AttributesFormatString=UDP Protocol [1997]
  RT2 : RateTransition  Commented=on  Integrity=off  OutPortSampleTime=1/100
  RT3 : RateTransition  Commented=on  Integrity=off  OutPortSampleTime=1/100
  Reshape : Reshape
  Scope{1..4} (4 alike) : Scope  Commented=on
  Scope5 : Scope
  Scope6 : Scope  NumInputPorts=2
  Scope7 : Scope
  Scope8 : Scope  NumInputPorts=2
  Scope9 : Scope
  Selector : Selector  InputPortWidth=3  IndexOptions=Index vector (dialog)  Indices=[3]  OutputSizes=1
  Selector1 : Selector  Commented=on  InputPortWidth=3  IndexOptions=Index vector (dialog)  Indices=[3 2 1]  OutputSizes=1
  Selector10 : Selector  InputPortWidth=12  IndexOptions=Index vector (dialog)  Indices=[1:6]  OutputSizes=1
  Selector11 : Selector  Commented=on  InputPortWidth=12  IndexOptions=Index vector (dialog)  Indices=[7:12]  OutputSizes=1
  Selector12 : Selector  InputPortWidth=6  IndexOptions=Index vector (dialog)  Indices=[4:6]  OutputSizes=1
  Selector13 : Selector  InputPortWidth=7  IndexOptions=Index vector (dialog)  Indices=[1:4]  OutputSizes=1
  Selector14 : Selector  InputPortWidth=7  IndexOptions=Index vector (dialog)  Indices=[5]  OutputSizes=1
  Selector15 : Selector  InputPortWidth=7  IndexOptions=Index vector (dialog)  Indices=[6,7]  OutputSizes=1
  Selector2 : Selector  Commented=on  InputPortWidth=12  IndexOptions=Index vector (dialog)  Indices=4:6  OutputSizes=1
  Selector3 : Selector  Commented=on  InputPortWidth=12  IndexOptions=Index vector (dialog)  Indices=10:12  OutputSizes=1
  Selector4 : Selector  Commented=on  InputPortWidth=12  IndexOptions=Index vector (dialog)  Indices=7:9  OutputSizes=1
  Selector5 : Selector  InputPortWidth=6  IndexOptions=Index vector (dialog)  Indices=[1:3]  OutputSizes=1
  Selector6 : Selector  InputPortWidth=6  IndexOptions=Index vector (dialog)  Indices=[4:6]  OutputSizes=1
  Selector7 : Selector  Commented=on  InputPortWidth=6  IndexOptions=Index vector (dialog)  Indices=[1:3]  OutputSizes=1
  Selector8 : Selector  Commented=on  InputPortWidth=6  IndexOptions=Index vector (dialog)  Indices=[4:6]  OutputSizes=1
  Selector9 : Selector  Commented=on  InputPortWidth=3  IndexOptions=Index vector (dialog)  Indices=[1]  OutputSizes=1
  Terminator1 : Terminator
  Vicon 2bodies data ready : Scope
  convert to mm : Gain  Gain=8190/65530
  convert to opti unit : Gain  Gain=400/65530
  convert to radian : Gain  Commented=on  Gain=2*pi/65530
  convert to radian1 : Gain  Gain=2/65530
  mm to m : Gain  Gain=0.001
  p_dot_cf : Scope  Commented=on
  raw_UDP : Scope  Commented=on
  vicon measure : Outport
  data ready : Outport  Port=2
  sensor : Outport  Port=3
  range_finder : Outport  Port=4
  optical_flow : Outport  Port=5
  wires:
  Gain5/1 -> Selector10/1
  Selector9/1 -> Goto22/1
  Discrete Derivative2/1 -> Goto13/1, p_dot_cf/1  "p_dot"
  Selector11/1 -> Selector8/1, Selector7/1
  RT3/1 -> Coordinate Transformation Conversion3/1
  Gain11/1 -> RT2/1
  Packet Input1/2 -> Vicon 2bodies data ready/1, data ready/1  "data ready"
  Digital Filter Design/1 -> Discrete Derivative2/1  "p"
  Selector6/1 -> Mux2/2
  Coordinate Transformation Conversion3/1 -> Selector9/1
  Selector5/1 -> Selector/1, Gain6/1
  Selector10/1 -> Selector6/1, Selector5/1
  Data Type Conversion1/1 -> Gain5/1
  Selector7/1 -> Gain11/1
  RT2/1 -> Goto3/1, Digital Filter Design/1
  Packet Input1/1 -> Data Type Conversion1/1
  Packet Input1/3 -> Terminator1/1  "data error"
  Selector8/1 -> RT3/1
  Add10/1 -> Mux2/1
  Constant40/1 -> Add10/2
  Gain6/1 -> Add10/1
  Mux2/1 -> vicon measure/1, Selector12/1
  Selector3/1 -> Gain3/1
  Gain7/1 -> Minus1/1
  Gain3/1 -> Minus2/1
  Gain1/1 -> Mux/2
  Selector1/1 -> convert to radian/1, Scope4/1  "sensor_raw_input"
  Constant1/1 -> Minus1/2
  Gain4/1 -> Mux/3
  Constant2/1 -> Minus2/2
  Selector2/1 -> Gain7/1
  Packet Input2/1 -> Data Type Conversion/1
  Demux/2 -> Gain1/1
  Gain2/1 -> Mux/1
  Minus2/1 -> Scope3/1
  Demux/3 -> Gain4/1
  Constant/1 -> Minus/2
  Data Type Conversion/1 -> Selector1/1
  Demux/1 -> Gain2/1
  Minus1/1 -> Scope1/1
  convert to radian/1 -> Minus/1
  Selector4/1 -> Demux/1
  Mux/1 -> Scope2/1
  Selector12/1 -> Scope6/1  "Vicon_EulXYZ"
  Gain8/1 -> Packet Output/1  "UDP uint16 3"
  Packet Input3/1 -> Data Type Conversion2/1, raw_UDP/1
  Constant3/1 -> Minus3/2
  convert to radian1/1 -> Minus3/1
  Minus3/1 -> Normalization/1  "sensor_EulXYZ"
  Packet Input3/2 -> Scope5/1
  Gain/1 -> sensor/1, Scope6/2
  Reshape/1 -> Scope7/1, Gain/1
  Normalization/1 -> Coordinate Transformation Conversion1/1
  Coordinate Transformation Conversion1/1 -> Reshape/1
  Constant4/1 -> ?
  Data Type Conversion2/1 -> Selector15/1, Selector14/1, Selector13/1
  Selector13/1 -> convert to radian1/1
  Selector14/1 -> convert to mm/1
  convert to mm/1 -> [range_finder], Add/1  "z (mm)"
  Selector/1 -> Scope8/1  "Vicon z (mm)"
  Add/1 -> Scope8/2
  Constant5/1 -> Add/2
  mm to m/1 -> range_finder/1
  [range_finder] -> mm to m/1
  Selector15/1 -> convert to opti unit/1
  convert to opti unit/1 -> Minus4/1  "opti x y"
  Constant6/1 -> Minus4/2
  Minus4/1 -> optical_flow/1, Scope9/1  "opti_xy"

== system opti_debug/archived ==
  note: Vicon Input (single rigid body) not in use
  Data Type Conversion : DataTypeConversion  Commented=on  OutDataTypeStr=double  SaturateOnIntegerOverflow=off  RndMeth=Floor
  Gain7 : Gain  Commented=on  Gain=1/mdl.vicon.gain
  Gain8 : Gain  Commented=on  Gain=0.001
  Goto9 : Goto  Commented=on  GotoTag=vicon_measure
  Mux : Mux  Commented=on  Inputs=2
  Packet Input : sldrtlib/Packet Input  Commented=on  SampleTime=1/2000  MaxMissedTicks=100  ShowMissedTicks=off  YieldWhenWaiting=off  DrvName=Standard_Devices/UDP_Protocol  DrvAddress=18000  DrvOptions=[0 18385 49 57 50 46 49 54 56 46 49 54 56 46 49 52 54 0 0 0 0 0 0 0 0 0 0 0 0 0 0 0 0 0 0 0 0 0 0 0 0 0 0 0 0 0 0 0 0 0 0 0 0 0 0 0 0 0 0 0 0 0 0 0 0 0 0 0 0 0 0 0 0 0 0 0 0 0 0 0 0 0 0 0 0 0 0 0 0 0 0 0 0 0 0 0 0 0 0 0 0 0 0 0 0 0 0 0 0 0 0 0 0 0 0 0 0 0 0 0 0 0 0 0 0 0 0 0 0 0 0 0 0 0 0 0 0 0 0 0 0 0 0 0 0 0 0 0 0 0 0 0 0 0 0 0 0 0 0 0 0 0 0 0 0 0 0 0 0 0 0 0 0 0 0 0 0 0 0 0 0 0 0 0 0 0 0 0 0 0 0 0 0 0 0 0 0 0 0 0 0 0 0 0 0 0 0 0 0 0 0 0 0 0 0 0 0 0 0 0 0 0 0 0 0 0 0 0 0 0 0 0 0 0 0 0 0 0 0 0 0 0 0 0 0 0 0 0 0 0 0 0 0 0 0 0]  PacketSize=24  DataTypes='6*int32'  ShowReady=on  ShowError=on  PacketID=1  ByteOrder=2  ShowTimestamp=off
      settings: AttributesFormatString=UDP Protocol [18000]
  Selector2 : Selector  Commented=on  InputPortWidth=6  IndexOptions=Index vector (dialog)  Indices=[1:3]  OutputSizes=1
  Selector3 : Selector  Commented=on  InputPortWidth=6  IndexOptions=Index vector (dialog)  Indices=[4:6]  OutputSizes=1
  Terminator11 : Terminator  Commented=on
  data ready : Scope  Commented=on
  wires:
  Packet Input/2 -> data ready/1  "data ready"
  Gain8/1 -> Mux/1
  Gain7/1 -> Selector3/1, Selector2/1
  Mux/1 -> Goto9/1
  Selector2/1 -> Gain8/1
  Data Type Conversion/1 -> Gain7/1
  Selector3/1 -> Mux/2
  Packet Input/3 -> Terminator11/1  "data error"
  Packet Input/1 -> Data Type Conversion/1

== system opti_debug/Archived data for rerun/time1 ==
  constant : Constant
  time : DiscreteIntegrator  gainval=mdl.f_high  InitialCondition=1  SampleTime=mdl.T_high  UpperSaturationLimit=1  LowerSaturationLimit=0  ICPrevOutput=DiscIntNeverNeededParam  ICPrevScaledInput=DiscIntNeverNeededParam
  index : Outport
  wires:
  constant/1 -> time/1
  time/1 -> index/1

== system opti_debug/Control scheme/Subsystem ==
  In1 : Inport
  Constant : Constant  Value=traj.en
  Constant1 : Constant  Value=ctr.rd_d_filt
  Digital Filter Design1 : dspfdesign/Digital Filter Design  mwdsp_browser_bugfix_var=off
  Scope : Scope  NumInputPorts=2
  Switch : Switch  Criteria=u2 > Threshold  Threshold=0.5  SaturateOnIntegerOverflow=off  InputSameDT=off
  Switch1 : Switch  Criteria=u2 > Threshold  Threshold=0.5  SaturateOnIntegerOverflow=off  InputSameDT=off
  Out1 : Outport
  wires:
  In1/1 -> Scope/1, Switch/1, Switch1/3, Digital Filter Design1/1
  Switch/1 -> Scope/2, Out1/1
  Constant/1 -> Switch/2
  Digital Filter Design1/1 -> Switch1/1
  Constant1/1 -> Switch1/2
  Switch1/1 -> Switch/3

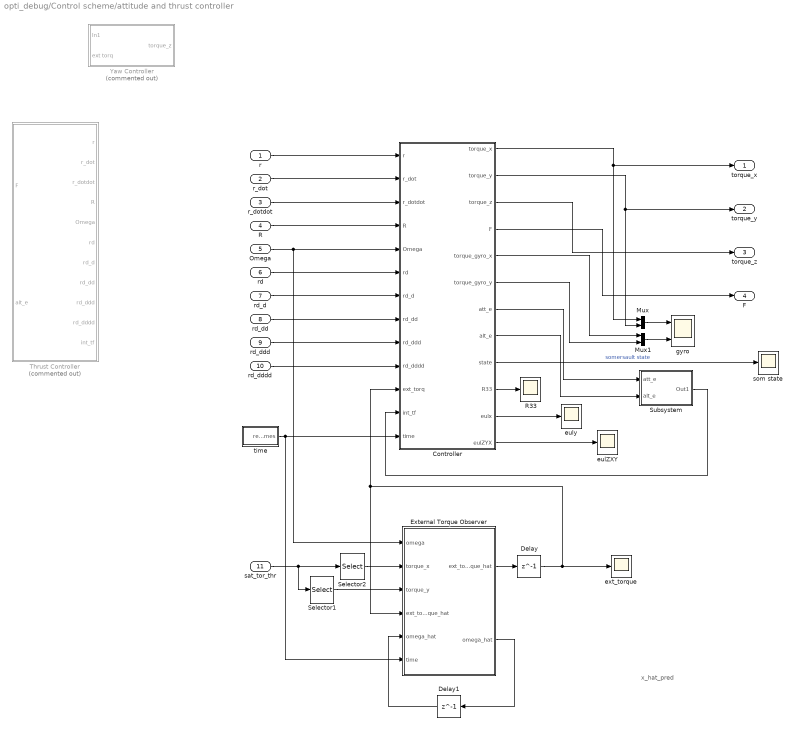
== system opti_debug/Control scheme/attitude and thrust controller ==
  note: x_hat_pred
  r : Inport
  r_dot : Inport  Port=2
  r_dotdot : Inport  Port=3
  R : Inport  Port=4
  Omega : Inport  Port=5
  rd : Inport  Port=6
  rd_d : Inport  Port=7
  rd_dd : Inport  Port=8
  rd_ddd : Inport  Port=9
  rd_dddd : Inport  Port=10
  sat_tor_thr : Inport  Port=11
  Controller : MATLAB Function  TreatAsAtomicUnit=on
  Delay : Delay  DelayLength=1  InitialCondition=ctr2.torque_obs.ext_torq_hat_init  SampleTime=mdl.T
  Delay1 : Delay  DelayLength=1  InitialCondition=ctr2.torque_obs.omega_hat_init  SampleTime=mdl.T
  External Torque Observer : MATLAB Function  TreatAsAtomicUnit=on
  Mux : Mux  Inputs=2
  Mux1 : Mux  Inputs=2
  R33 : Scope
  Selector1 : Selector  InputPortWidth=4  IndexOptions=Index vector (dialog)  Indices=[2]  OutputSizes=1
  Selector2 : Selector  InputPortWidth=4  IndexOptions=Index vector (dialog)  Indices=[1]  OutputSizes=1
  Subsystem : Subsystem
  Thrust Controller : MATLAB Function  Commented=on  TreatAsAtomicUnit=on
  Yaw Controller : Subsystem  Commented=on
  eulZXY : Scope
  euly : Scope
  ext_torque : Scope
  gyro : Scope  NumInputPorts=2
  som state : Scope
  time : Subsystem
  torque_x : Outport
  torque_y : Outport  Port=2
  torque_z : Outport  Port=3
  F : Outport  Port=4
  wires:
  r/1 -> Controller/1(r)
  Controller/1(torque_x) -> torque_x/1, Mux/1
  r_dot/1 -> Controller/2(r_dot)
  r_dotdot/1 -> Controller/3(r_dotdot)
  R/1 -> Controller/4(R)
  Controller/2(torque_y) -> torque_y/1, Mux/2
  Omega/1 -> External Torque Observer/1(omega), Controller/5(Omega)
  rd/1 -> Controller/6(rd)
  rd_d/1 -> Controller/7(rd_d)
  rd_dd/1 -> Controller/8(rd_dd)
  rd_ddd/1 -> Controller/9(rd_ddd)
  rd_dddd/1 -> Controller/10(rd_dddd)
  Controller/3(torque_z) -> torque_z/1
  External Torque Observer/2(omega_hat) -> Delay1/1
  Delay/1 -> ext_torque/1, External Torque Observer/4("ext_torque_hat "), Controller/11(ext_torq)
  External Torque Observer/1(ext_torque_hat) -> Delay/1
  Delay1/1 -> External Torque Observer/5("omega_hat ")
  time/1(real times) -> External Torque Observer/6(time), Controller/13(time)
  Subsystem/1(Out1) -> Controller/12(int_tf)
  Controller/7(att_e) -> Subsystem/1(att_e)
  Selector2/1 -> External Torque Observer/2(torque_x)
  Selector1/1 -> External Torque Observer/3(torque_y)
  sat_tor_thr/1 -> Selector2/1, Selector1/1
  Controller/8(alt_e) -> Subsystem/2(alt_e)
  Controller/4(F) -> F/1
  Mux/1 -> gyro/1
  Mux1/1 -> gyro/2
  Controller/5(torque_gyro_x) -> Mux1/1
  Controller/12(eulZYX) -> eulZXY/1
  Controller/6(torque_gyro_y) -> Mux1/2
  Controller/9(state) -> som state/1  "somersault state"
  Controller/11(eulx) -> euly/1
  Controller/10(R33) -> R33/1

== system opti_debug/Control scheme/observer ==
  xyz : Inport
  euler : Inport  Port=2
  Rotaion : Subsystem
  lateral observer : Subsystem
  r : Outport
  r_dot : Outport  Port=2
  r_dotdot : Outport  Port=3
  R : Outport  Port=4
  Omega : Outport  Port=5
  Rdot : Outport  Port=6
  wires:
  lateral observer/1(r) -> r/1
  xyz/1 -> lateral observer/1(XYZ)
  lateral observer/2(r_dot) -> r_dot/1
  lateral observer/3(r_dotdot) -> r_dotdot/1
  Rotaion/1(R) -> R/1
  euler/1 -> Rotaion/1(Euler)
  Rotaion/2(Rdot) -> Rdot/1
  Rotaion/3(Omega) -> Omega/1

== system opti_debug/Control scheme/time ==
  constant : Constant
  time : DiscreteIntegrator  gainval=1  SampleTime=-1  UpperSaturationLimit=1  LowerSaturationLimit=0  ICPrevOutput=DiscIntNeverNeededParam  ICPrevScaledInput=DiscIntNeverNeededParam
  real times : Outport
  wires:
  constant/1 -> time/1
  time/1 -> real times/1

== system opti_debug/Motor thrust to voltage mapping/Subsystem ==
  In1 : Inport
  Constant8 : Constant
  Constant9 : Constant  Value=rsim.en | ctr.elec_cehck
  Data Type Conversion1 : DataTypeConversion  SaturateOnIntegerOverflow=off  RndMeth=Floor
  MATLAB Function : MATLAB Function  TreatAsAtomicUnit=on
  Switch2 : Switch  Criteria=u2 > Threshold  SaturateOnIntegerOverflow=off  InputSameDT=off
  Zero-Order Hold6 : ZeroOrderHold  SampleTime=mdl.T
  time : Subsystem
  times1 : Product  RndMeth=Zero
  Out1 : Outport
  wires:
  Constant9/1 -> Switch2/2
  Switch2/1 -> times1/1
  Constant8/1 -> Data Type Conversion1/1
  time/1(real times) -> MATLAB Function/1(t)
  times1/1 -> Zero-Order Hold6/1
  MATLAB Function/1(enable) -> times1/2
  In1/1 -> Switch2/3
  Data Type Conversion1/1 -> Switch2/1
  Zero-Order Hold6/1 -> Out1/1
